simulink model "Corrected"  (R2020a)
settings: Solver=VariableStepAuto  StartTime=0.0  StopTime=10.0  RelTol=1e-3  EnableMultiTasking=on
undefined symbols (not defined in the file): X, Y, Z
libraries: sm_lib x47, nesl_utility x10
(part 2 of 2)

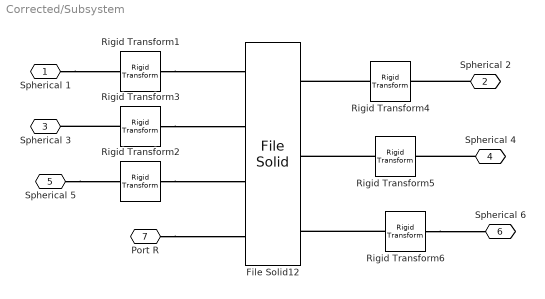
== system Corrected/Subsystem ==
  File Solid12 : sm_lib/Body Elements/File Solid  ExtGeomFileName=F:\JATC\Simulation\Parallel Robot\CAD Files\Upper_Base_New.sat  UnitType=FromFile  ExtGeomFileUnits=m  StepReaderType=HEX  ExportConvexHullGeometry=off  InertiaType=CalculateFromGeometry  Mass=1  MassUnits=kg  CenterOfMass=[0 0 0]  CenterOfMassUnits=m  MomentsOfInertia=[1 1 1]  MomentsOfInertiaUnits=kg*m^2  ProductsOfInertia=[0 0 0]  ProductsOfInertiaUnits=kg*m^2  BasedOnType=Density  Density=1000  DensityUnits=kg/m^3  DoExposeReferenceFrame=off  SerializedFrames=<Frames><Frame><Id>Frame1</Id><Value><Name>F1</Name><Origin><Source>GeometricFeature</Source><FeatureName>circular curve 142</FeatureName></Origin><PrimaryAxis><DefinedDirection>+Z</DefinedDirection><Source>ReferenceFrame</Source><SourceDirection>+Z</SourceDirection><FeatureName></FeatureName></PrimaryAxis><SecondaryAxis><DefinedDirection>+X</DefinedDirection><Source>ReferenceFrame</Source><SourceDirection>+X</SourceDirection><FeatureName></FeatureName></SecondaryAxis></Value></Frame><Frame><Id>Frame2</Id><Value><Name>F2</Name><Origin><Source>GeometricFeature</Source><FeatureName>circular curve 349</FeatureName></Origin><PrimaryAxis><DefinedDirection>+Z</DefinedDirection><Source>ReferenceFrame</Source><SourceDirection>+Z</SourceDirection><FeatureName></FeatureName></PrimaryAxis><SecondaryAxis><DefinedDirection>+X</DefinedDirection><Source>ReferenceFrame</Source><SourceDirection>+X</SourceDirection><FeatureName></FeatureName></SecondaryAxis></Value></Frame><Frame><Id>Frame3</Id><Value><Name>F3</Name><Origin><Source>GeometricFeature</Source><FeatureName>circular curve 4</FeatureName></Origin><PrimaryAxis><DefinedDirection>+Z</DefinedDirection><Source>ReferenceFrame</Source><SourceDirection>+Z</SourceDirection><FeatureName></FeatureName></PrimaryAxis><SecondaryAxis><DefinedDirection>+X</DefinedDirection><Source>ReferenceFrame</Source><SourceDirection>+X</SourceDirection><FeatureName></FeatureName></SecondaryAxis></Value></Frame><Frame><Id>Frame4</Id><Value><Name>F4</Name><Origin><Source>GeometricFeature</Source><FeatureName>circular curve 211</FeatureName></Origin><PrimaryAxis><DefinedDirection>+Z</DefinedDirection><Source>ReferenceFrame</Source><SourceDirection>+Z</SourceDirection><FeatureName></FeatureName></PrimaryAxis><SecondaryAxis><DefinedDirection>+X</DefinedDirection><Source>ReferenceFrame</Source><SourceDirection>+X</SourceDirection><FeatureName></FeatureName></SecondaryAxis></Value></Frame><Frame><Id>Frame5</Id><Value><Name>F5</Name><Origin><Source>GeometricFeature</Source><FeatureName>circular curve 73</FeatureName></Origin><PrimaryAxis><DefinedDirection>+Z</DefinedDirection><Source>ReferenceFrame</Source><SourceDirection>+Z</SourceDirection><FeatureName></FeatureName></PrimaryAxis><SecondaryAxis><DefinedDirection>+X</DefinedDirection><Source>ReferenceFrame</Source><SourceDirection>+X</SourceDirection><FeatureName></FeatureName></SecondaryAxis></Value></Frame><Frame><Id>Frame6</Id><Value><Name>F6</Name><Origin><Source>GeometricFeature</Source><FeatureName>circular curve 280</FeatureName></Origin><PrimaryAxis><DefinedDirection>+Z</DefinedDirection><Source>ReferenceFrame</Source><SourceDirection>+Z</SourceDirection><FeatureName></FeatureName></PrimaryAxis><SecondaryAxis><DefinedDirection>+X</DefinedDirection><Source>ReferenceFrame</Source><SourceDirection>+X</SourceDirection><FeatureName></FeatureName></SecondaryAxis></Value></Frame><Frame><Id>Frame7</Id><Value><Name>F7</Name><Origin><Source>ReferenceFrame</Source><FeatureName></FeatureName></Origin><PrimaryAxis><DefinedDirection>+Z</DefinedDirection><Source>ReferenceFrame</Source><SourceDirection>+Z</SourceDirection><FeatureName></FeatureName></PrimaryAxis><SecondaryAxis><DefinedDirection>+X</DefinedDirection><Source>ReferenceFrame</Source><SourceDirection>+X</SourceDirection><FeatureName></FeatureName></SecondaryAxis></Value></Frame></Frames>  GraphicType=FromGeometry  MarkerShape=Sphere  MarkerSize=10  GraphicVisPropType=SimpleVisualProperties  GraphicDiffuseColor=[0.8 0.0 0.2]  GraphicSpecularColor=[0.5 0.5 0.5 1.0]  GraphicAmbientColor=[0.15 0.15 0.15 1.0]  GraphicEmissiveColor=[0.0 0.0 0.0 1.0]  GraphicShininess=75  GraphicOpacity=1.0
  Rigid Transform{1..6} (6 alike) : sm_lib/Frames and Transforms/Rigid Transform  TranslationMethod=StandardAxis  TranslationStandardOffset=2.027  TranslationLengthUnit=mm  TranslationStandardAxis=-Z  TranslationCartesianOffset=[0 0 0]  TranslationROffset=0  TranslationROffsetUnits=m  TranslationZOffset=0  TranslationZOffsetUnits=m  TranslationThetaOffset=0  TranslationThetaOffsetUnits=deg  RotationMethod=None  RotationAngleUnits=deg  RotationStandardAxis=+Z  RotationAngle=0.0  RotationArbitraryAxis=[0 0 1]  FollAlignAxisA=+X  BaseAlignAxisA=+Y  FollAlignAxisB=+Y  BaseAlignAxisB=+Z  RotationSequenceAxes=FollowerAxes  RotationSequence=XYX  RotationSequenceAngles=[0 0 0]  RotationSequenceAnglesUnits=deg  RotationMatrix=[1 0 0; 0 1 0; 0 0 1]
  Spherical 1 : PMIOPort  Side=Left
  Spherical 2 : PMIOPort  Port=2  Side=Left
  Spherical 3 : PMIOPort  Port=3  Side=Left
  Spherical 4 : PMIOPort  Port=4  Side=Left
  Spherical 5 : PMIOPort  Port=5  Side=Left
  Spherical 6 : PMIOPort  Port=6  Side=Left
  Port R : PMIOPort  Port=7  Side=Right
  connections:
  Spherical 2/RConn1 -- Rigid Transform4/RConn1
  Rigid Transform3/RConn1 -- Spherical 3/RConn1
  Spherical 4/RConn1 -- Rigid Transform5/RConn1
  Spherical 5/RConn1 -- Rigid Transform2/RConn1
  Rigid Transform6/RConn1 -- Spherical 6/RConn1
  Spherical 1/RConn1 -- Rigid Transform1/RConn1
  Rigid Transform1/LConn1 -- File Solid12/LConn1
  Rigid Transform4/LConn1 -- File Solid12/RConn1
  Rigid Transform3/LConn1 -- File Solid12/LConn2
  Rigid Transform5/LConn1 -- File Solid12/RConn2
  Rigid Transform2/LConn1 -- File Solid12/LConn3
  Rigid Transform6/LConn1 -- File Solid12/RConn3
  Port R/RConn1 -- File Solid12/LConn4

== matlab function Corrected/MATLAB Function ==
  data: x input; l1 output; y input; z input; alp input; bet input; gma input; l2 output; l3 output; l4 output; l5 output; l6 output
function [l1, l2, l3, l4, l5, l6] = IK(x, y, z, alp, bet, gma)
pt = zeros(6,3);
pb = zeros(6,3);
ptg = zeros(6,3);
vec = zeros(6,3);
l = zeros(6,1);


% // Inverse kinematics of the Stewart platform manipulator
% // For a given pose of the moving platform what will be the required leg lengths

gm=[270-22.5,270+22.5,30-22.5,30+22.5,150-22.5,150+22.5]*(pi/180);
for i = 1:6
    pt(i,1:3) = rtz(gm(i))*[0.090,0,0]';
end

gm1=[210+17,330-17,330+17,90-17,90+17,210-17]*(pi/180);
for i = 1:6
    pb(i,1:3) = rtz(gm1(i))*[0.120,0,0]';
end

for i = 1:6
    ptg(i,1:3) = [x y z]'+ rtz(gm(i))*[0.090,0,0]';
end

for i = 1:6
    vec(i,1:3) = ptg(i,1:3)-pb(i,1:3);
    l(i)= sqrt(dot(vec(i,1:3),vec(i,1:3)));
end

function rz = rtz(gm)
    rz = [cos(gm) -sin(gm) 0; sin(gm) cos(gm) 0; 0 0 1];
end

l1 = l(1);
l2 = l(2);
l3 = l(3);
l4 = l(4);
l5 = l(5);
l6 = l(6);

end
